simulink model "piezo"  (R2014b)
settings: Solver=ode45  StartTime=0.0  StopTime=0.02  MaxStep=0.00001  MinStep=0.000001  RelTol=1e-3
values from neighbouring files (symbols this model uses):
  Cp = 0.8*10^8    (= 80000000)    [parametrs.m]
  Fb = 50    [parametrs.m]
  Kd = 1.1*10^3    (= 1100)    [parametrs.m]
  Ko = 8.2    [parametrs.m]
  Ku = Upm/Um    (= 55)    [parametrs.m]
  Kx = 1/0.002    (= 500)    [parametrs.m]
  Ky = 2    [parametrs.m]
  m = 0.3    [parametrs.m]
  r = 1/0.005    (= 200)    [parametrs.m]
  Tu = 0.05/1000    (= 5e-05)    [parametrs.m]
libraries: simulink x2
settings Model: Creator=Игорь  LastModifiedBy=Игорь

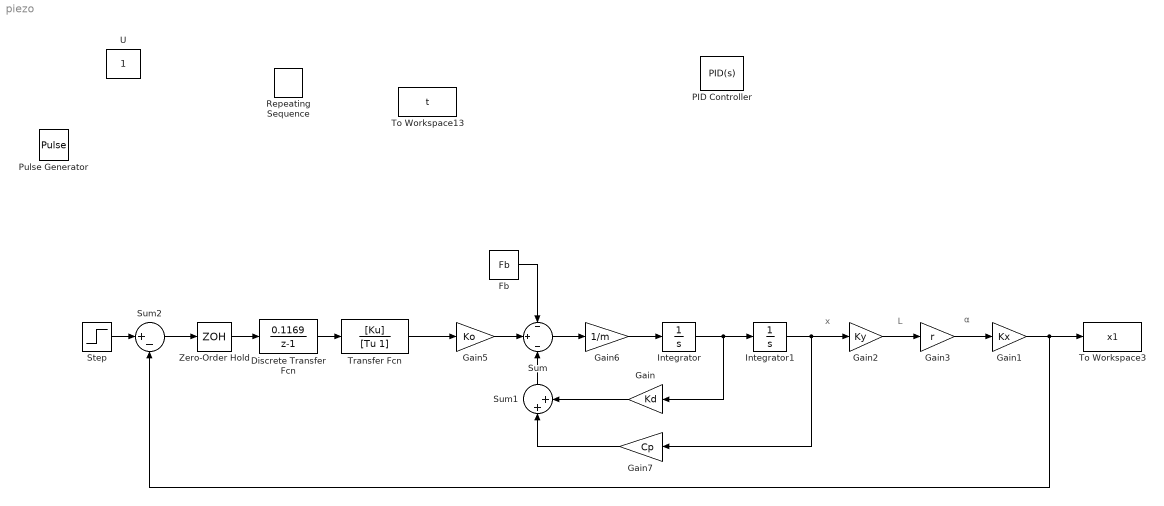
== system piezo ==
  note: α
  note: L
  note: x
  Discrete Transfer Fcn : DiscreteTransferFcn  Numerator=[0.1169]  Denominator=[1 -1]
  Fb : Constant  Value=Fb
  Gain : Gain  Gain=Kd
  Gain1 : Gain  Gain=Kx
  Gain2 : Gain  Gain=Ky
  Gain3 : Gain  Gain=r
  Gain5 : Gain  Gain=Ko
  Gain6 : Gain  Gain=1/m
  Gain7 : Gain  Gain=Cp
  Integrator : Integrator
  Integrator1 : Integrator
  PID Controller : simulink/Continuous/PID Controller  Controller=PID  TimeDomain=Continuous-time  SampleTime=-1  IntegratorMethod=Forward Euler  FilterMethod=Forward Euler  Form=Parallel  P=0  I=1168.59747755308  D=0  N=100  InitialConditionSource=internal  InitialConditionForIntegrator=0  InitialConditionForFilter=0  ExternalReset=none  LimitOutput=off  UpperSaturationLimit=inf  LowerSaturationLimit=-inf  LinearizeAsGain=on  AntiWindupMode=none  Kb=1  TrackingMode=off  Kt=1  PParamMin=[]  PParamMax=[]  IParamMin=[]  IParamMax=[]  DParamMin=[]  DParamMax=[]  NParamMin=[]  NParamMax=[]  KbParamMin=[]  KbParamMax=[]  KtParamMin=[]  KtParamMax=[]  POutMin=[]  POutMax=[]  IOutMin=[]  IOutMax=[]  DOutMin=[]  DOutMax=[]  NOutMin=[]  NOutMax=[]  KbOutMin=[]  KbOutMax=[]  KtOutMin=[]  KtOutMax=[]  IntegratorOutMin=[]  IntegratorOutMax=[]  FilterOutMin=[]  FilterOutMax=[]  SumOutMin=[]  SumOutMax=[]  SumI1OutMin=[]  SumI1OutMax=[]  SumI2OutMin=[]  SumI2OutMax=[]  SumI3OutMin=[]  SumI3OutMax=[]  SumDOutMin=[]  SumDOutMax=[]  SaturationOutMin=[]  SaturationOutMax=[]  IntegratorContinuousStateAttributes=''  IntegratorStateMustResolveToSignalObject=off  IntegratorRTWStateStorageClass=Auto  FilterContinuousStateAttributes=''  FilterStateMustResolveToSignalObject=off  FilterRTWStateStorageClass=Auto  DifferentiatorICPrevScaledInput=0  DifferentiatorOutMin=[]  DifferentiatorOutMax=[]  UseFilter=on
  Pulse Generator : DiscretePulseGenerator  PulseType=Time based  Period=0.0001  PulseWidth=50
  Repeating Sequence : simulink/Sources/Repeating Sequence  rep_seq_t=[0 0.00001]  rep_seq_y=[0 1]
  Step : Step  Time=0  SampleTime=0
  Sum : Sum  Inputs=-|+|-
  Sum1 : Sum  Inputs=|++
  Sum2 : Sum  Inputs=|+-
  To Workspace13 : ToWorkspace  VariableName=t  SaveFormat=Timeseries  SampleTime=-1
  To Workspace3 : ToWorkspace  VariableName=x1  SaveFormat=Timeseries  SampleTime=-1
  Transfer Fcn : TransferFcn  Numerator=[Ku]  Denominator=[Tu 1]
  U : Constant
  Zero-Order Hold : ZeroOrderHold  SampleTime=0.0001
  wires:
  Gain5/1 -> Sum/2
  Integrator/1 -> Integrator1/1, Gain/1
  Gain6/1 -> Integrator/1
  Sum/1 -> Gain6/1
  Gain/1 -> Sum1/2
  Sum1/1 -> Sum/3
  Gain7/1 -> Sum1/1
  Fb/1 -> Sum/1
  Integrator1/1 -> Gain2/1, Gain7/1
  Zero-Order Hold/1 -> Discrete Transfer Fcn/1
  Gain2/1 -> Gain3/1
  Gain3/1 -> Gain1/1
  Gain1/1 -> Sum2/2, To Workspace3/1
  Transfer Fcn/1 -> Gain5/1
  Discrete Transfer Fcn/1 -> Transfer Fcn/1
  Step/1 -> Sum2/1
  Sum2/1 -> Zero-Order Hold/1
